simulink model "ch6example7"  (Simulink 5.0)
settings: Solver=FixedStepDiscrete  StartTime=0.0  StopTime=10.0  FixedStep=1/8000  RelTol=1e-3
libraries: commutil2 x2
settings Model: LastModifiedBy=shaoyubin

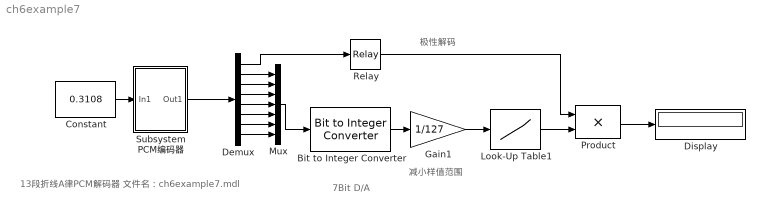
== system ch6example7 ==
  note: 13段折线A律PCM解码器
      | 文件名：ch6example7.mdl
  note: 极性解码
  note: 7Bit D/A
  note: 减小样值范围
  Bit to Integer Converter : commutil2/Bit to Integer Converter  nbits=7
  Constant : Constant  Value=0.3108
  Demux : Demux  Outputs=8
  Display : Display
  Gain1 : Gain  Gain=1/127  SaturateOnIntegerOverflow=on
  Look-Up Table1 : Lookup  InputValues=[0:1/8:1]  OutputValues=[0,1/128,1/64,1/32,1/16,1/8,1/4,1/2,1]  SaturateOnIntegerOverflow=on
  Mux : Mux  Inputs=7
  Product : Product  SaturateOnIntegerOverflow=on
  Relay : Relay  OnSwitchValue=0.5  OffSwitchValue=0.5  OffOutputValue=-1
  Subsystem PCM编码器 : Subsystem
  wires:
  Constant/1 -> Subsystem PCM编码器/1(In1)
  Bit to Integer Converter/1 -> Gain1/1
  Look-Up Table1/1 -> Product/2
  Relay/1 -> Product/1
  Product/1 -> Display/1
  Subsystem PCM编码器/1(Out1) -> Demux/1
  Mux/1 -> Bit to Integer Converter/1
  Demux/1 -> Relay/1
  Demux/2 -> Mux/1
  Demux/3 -> Mux/2
  Demux/8 -> Mux/7
  Demux/7 -> Mux/6
  Demux/6 -> Mux/5
  Demux/5 -> Mux/4
  Demux/4 -> Mux/3
  Gain1/1 -> Look-Up Table1/1

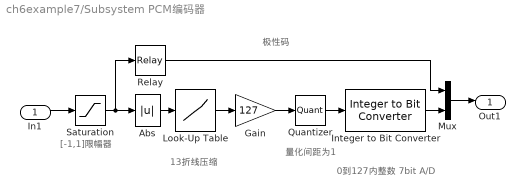
== system ch6example7/Subsystem PCM编码器 ==
  note: 0到127内整数
      | 7bit A/D
  note: [-1,1]限幅器
  note: 极性码
  note: 13折线压缩
  note: 量化间距为1
  In1 : Inport
  Abs : Abs  SaturateOnIntegerOverflow=on
  Gain : Gain  Gain=127  SaturateOnIntegerOverflow=on
  Integer to Bit Converter : commutil2/Integer to Bit Converter  nbits=7
  Look-Up Table : Lookup  InputValues=[-1,-1/2,-1/4,-1/8,-1/16,-1/32,-1/64,-1/128,0,1/128,1/64,1/32,1/16,1/8,1/4,1/2,1]  OutputValues=[-1:1/8:1]  SaturateOnIntegerOverflow=on
  Mux : Mux  Inputs=2
  Quantizer : Quantizer  QuantizationInterval=1
  Relay : Relay
  Saturation : Saturate  UpperLimit=1  LowerLimit=-1
  Out1 : Outport
  wires:
  Look-Up Table/1 -> Gain/1
  Quantizer/1 -> Integer to Bit Converter/1
  Gain/1 -> Quantizer/1
  Abs/1 -> Look-Up Table/1
  Relay/1 -> Mux/1
  Integer to Bit Converter/1 -> Mux/2
  Saturation/1 -> Abs/1, Relay/1
  Mux/1 -> Out1/1
  In1/1 -> Saturation/1
